simulink model "longmendiao_2"  (R2022b)
settings: Solver=VariableStepAuto  StartTime=0.0  StopTime=100  RelTol=1e-3
settings Model: Creator=MasterMo  LastModifiedBy=47800
settings SolverCC: AlgebraicLoopSolver=TrustRegion
settings DebuggingCC: UnconnectedInputMsg=warning  UnconnectedOutputMsg=warning  UnconnectedLineMsg=warning  SFMachineParentedDataDiag=warning
settings ModelReferenceCC: EnableRefExpFcnMdlSchedulingChecks=on

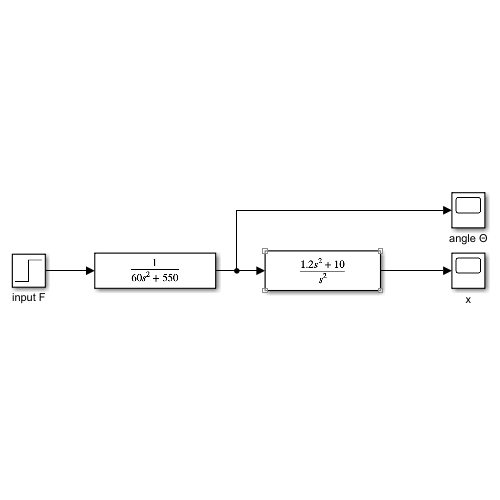
[thumbnail: Simulink's stored preview of the top-level diagram]
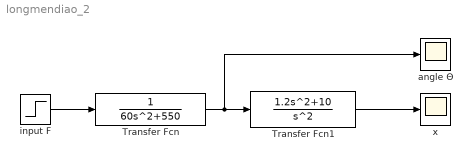
== system longmendiao_2 ==
  Transfer Fcn : TransferFcn  Denominator=[60 0 550]
  Transfer Fcn1 : TransferFcn  Numerator=[1.2 0 10]  Denominator=[1 0 0]
  angle Θ : Scope
  input F : Step  After=2  SampleTime=0
  x : Scope
  wires:
  input F/1 -> Transfer Fcn/1
  Transfer Fcn1/1 -> x/1
  Transfer Fcn/1 -> angle Θ/1, Transfer Fcn1/1
